simulink library "SingleMotor_Duty_to_inc"  (R2015a)
settings: Solver=ode45  StartTime=0.0  StopTime=10.0  RelTol=1e-3
undefined symbols (not defined in the file): EncRes, FreqTriangle, TsEnc, Ubus
libraries: simulink x1, powerlib_meascontrol x1
settings Model: Creator=tbaroche  LastModifiedBy=tbaroche

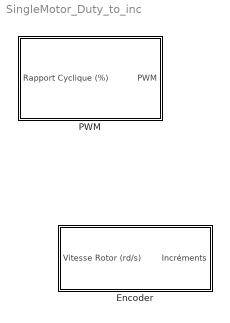
== system SingleMotor_Duty_to_inc ==
  Encoder : Subsystem  mask{EncRes=EncRes}
      mask prompts: EncRes "Résolution de l'encodeur (inc/tr)"
  PWM : Subsystem  mask{FreqTriangle=FreqTriangle}
      mask prompts: FreqTriangle "Fréquence du PWM (Hz)"

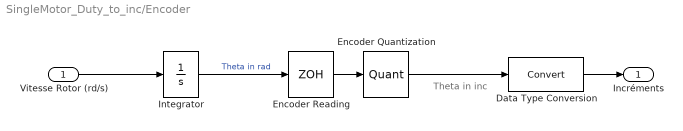
== system SingleMotor_Duty_to_inc/Encoder ==
  note: Theta in inc
  Vitesse Rotor (rd/s) : Inport
  Data Type Conversion : DataTypeConversion
  Encoder Quantization : Quantizer  QuantizationInterval=(2*pi)/EncRes
  Encoder Reading : ZeroOrderHold  SampleTime=TsEnc
  Integrator : Integrator
  Incréments : Outport
  wires:
  Integrator/1 -> Encoder Reading/1  "Theta in rad"
  Vitesse Rotor (rd/s)/1 -> Integrator/1
  Data Type Conversion/1 -> Incréments/1
  Encoder Reading/1 -> Encoder Quantization/1
  Encoder Quantization/1 -> Data Type Conversion/1

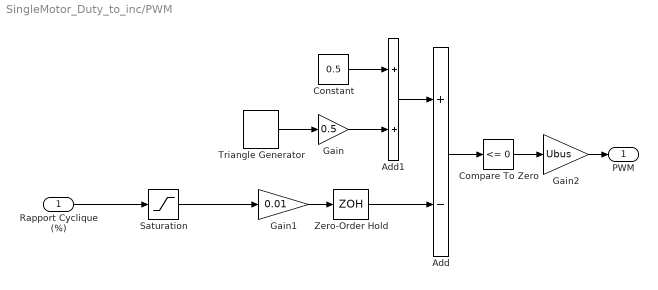
== system SingleMotor_Duty_to_inc/PWM ==
  Rapport Cyclique (%) : Inport
  Add : Sum  Inputs=+-
  Add1 : Sum
  Compare To Zero : simulink/Logic and Bit Operations/Compare To Zero  relop=<=  OutDataTypeStr=boolean
  Constant : Constant  Value=0.5
  Gain : Gain  Gain=0.5
  Gain1 : Gain  Gain=0.01
  Gain2 : Gain  Gain=Ubus  OutDataTypeStr=double
  Saturation : Saturate  UpperLimit=100  LowerLimit=-100
  Triangle Generator : powerlib_meascontrol/Pulse & Signal Generators/Triangle Generator  Freq=FreqTriangle  Phase=90  Ts=0
  Zero-Order Hold : ZeroOrderHold
  PWM : Outport
  wires:
  Constant/1 -> Add1/1
  Gain/1 -> Add1/2
  Zero-Order Hold/1 -> Add/2
  Rapport Cyclique (%)/1 -> Saturation/1
  Triangle Generator/1 -> Gain/1
  Compare To Zero/1 -> Gain2/1
  Add1/1 -> Add/1
  Add/1 -> Compare To Zero/1
  Gain1/1 -> Zero-Order Hold/1
  Gain2/1 -> PWM/1
  Saturation/1 -> Gain1/1
